simulink model "CurrentSensor"  (R2023a)
settings: Solver=VariableStepAuto  StartTime=0.0  StopTime=10.0  RelTol=1e-3
settings Model: Creator=Сафроновы  LastModifiedBy=Сафроновы

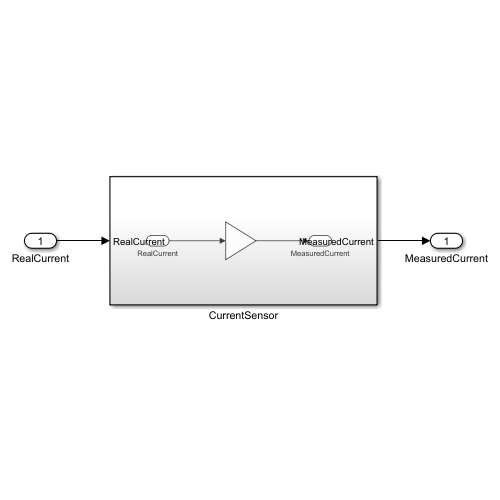
[thumbnail: Simulink's stored preview of the top-level diagram]
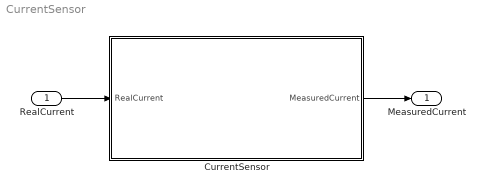
== system CurrentSensor ==
  RealCurrent : Inport
  CurrentSensor : Subsystem
  MeasuredCurrent : Outport
  wires:
  RealCurrent/1 -> CurrentSensor/1(RealCurrent)
  CurrentSensor/1(MeasuredCurrent) -> MeasuredCurrent/1

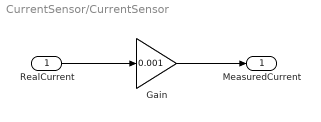
== system CurrentSensor/CurrentSensor ==
  RealCurrent : Inport
  Gain : Gain  Gain=0.001
  MeasuredCurrent : Outport
  wires:
  Gain/1 -> MeasuredCurrent/1
  RealCurrent/1 -> Gain/1
